simulink model "cascade_model"  (R2026a)
settings: Solver=VariableStepAuto  StopTime=75
values from neighbouring files (symbols this model uses):
  params = base    [build_params.m]    (also in determine_cost.m = build_params(struct(      'm_structure', m,      'x_thrust',; run_initial.m = rig())
undefined symbols (not defined in the file or in its folder): DiscIntNeverNeededParam
settings Model: Creator=hardik-karan  LastModifiedBy=Work

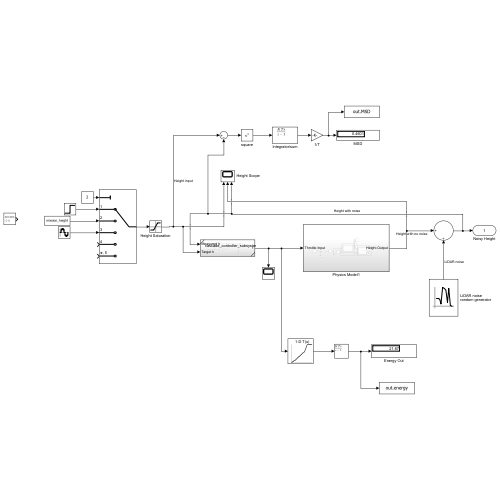
[thumbnail: Simulink's stored preview of the top-level diagram]
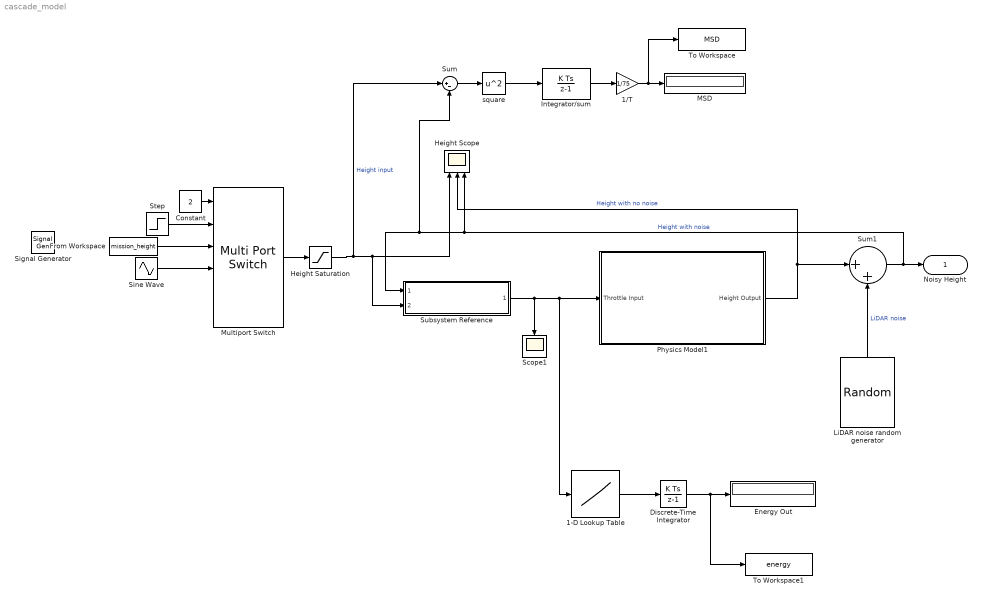
== system cascade_model ==
  1-D Lookup Table : Lookup_n-D  NumberOfTableDimensions=1  BreakpointsForDimension1=params.throttle_grid  Table=params.power_grid  InternalRulePriority=Speed  RndMeth=Simplest
  1/T : Gain  Gain=1/75
  Constant : Constant  Value=2
  Discrete-Time Integrator : DiscreteIntegrator  gainval=0.001  SampleTime=params.dt  ICPrevOutput=DiscIntNeverNeededParam  ICPrevScaledInput=DiscIntNeverNeededParam
  Energy Out : Display
      settings: Decimation=3
  From Workspace : FromWorkspace  VariableName=mission_height  SampleTime=params.dt  OutputAfterFinalValue=Holding final value
  Height Saturation : Saturate  UpperLimit=1.44  LowerLimit=0
  Height Scope : Scope  NumInputPorts=3
      settings: ActiveDisplayYMinimum=-4.73003641066337  ActiveDisplayYMaximum=6.0208709311882966  DataLoggingVariableName=ScopeData2
  Integrator/sum : DiscreteIntegrator  SampleTime=-1  ICPrevOutput=DiscIntNeverNeededParam  ICPrevScaledInput=DiscIntNeverNeededParam
  LiDAR noise random generator : RandomNumber  Variance=4.913e-05  SampleTime=params.dt
  MSD : Display
      settings: Decimation=6
  Multiport Switch : MultiPortSwitch  Inputs=5  SaturateOnIntegerOverflow=off  InputSameDT=off
  Physics Model1 : Subsystem
  Scope1 : Scope
      settings: ActiveDisplayYMinimum=-9.9999999999999982  ActiveDisplayYMaximum=90  DataLoggingVariableName=ScopeData4
  Signal Generator : SignalGenerator  Units=rad/sec
  Sine Wave : Sin  Amplitude=0.5  Bias=0.5  SampleTime=params.dt
  Step : Step  FinalValue=0.5  SampleTime=0
  Subsystem Reference : Subsystem  ReferencedSubsystem=cascade_controller_subsystem
  Sum : Sum  Inputs=|+-
  Sum1 : Sum  Inputs=|++
  To Workspace : ToWorkspace  VariableName=MSD  SaveFormat=Timeseries  SampleTime=-1
  To Workspace1 : ToWorkspace  VariableName=energy  SaveFormat=Timeseries  SampleTime=-1
  square : Math  Operator=square
  Noisy Height : Outport
  wires:
  Multiport Switch/1 -> Height Saturation/1
  Subsystem Reference/1 -> 1-D Lookup Table/1, Physics Model1/1(Throttle Input), Scope1/1
  Height Saturation/1 -> Sum/1, Subsystem Reference/2, Height Scope/1  "Height input"
  Physics Model1/1(Height Output) -> Height Scope/2, Sum1/1  "Height with no noise"
  Step/1 -> Multiport Switch/2
  Constant/1 -> Multiport Switch/1
  From Workspace/1 -> Multiport Switch/3
  Integrator/sum/1 -> 1/T/1
  1/T/1 -> To Workspace/1, MSD/1
  square/1 -> Integrator/sum/1
  Sum/1 -> square/1
  LiDAR noise random generator/1 -> Sum1/2  "LiDAR noise"
  Sum1/1 -> Subsystem Reference/1, Sum/2, Height Scope/3, Noisy Height/1  "Height with noise"
  1-D Lookup Table/1 -> Discrete-Time Integrator/1
  Discrete-Time Integrator/1 -> To Workspace1/1, Energy Out/1
  Sine Wave/1 -> Multiport Switch/4

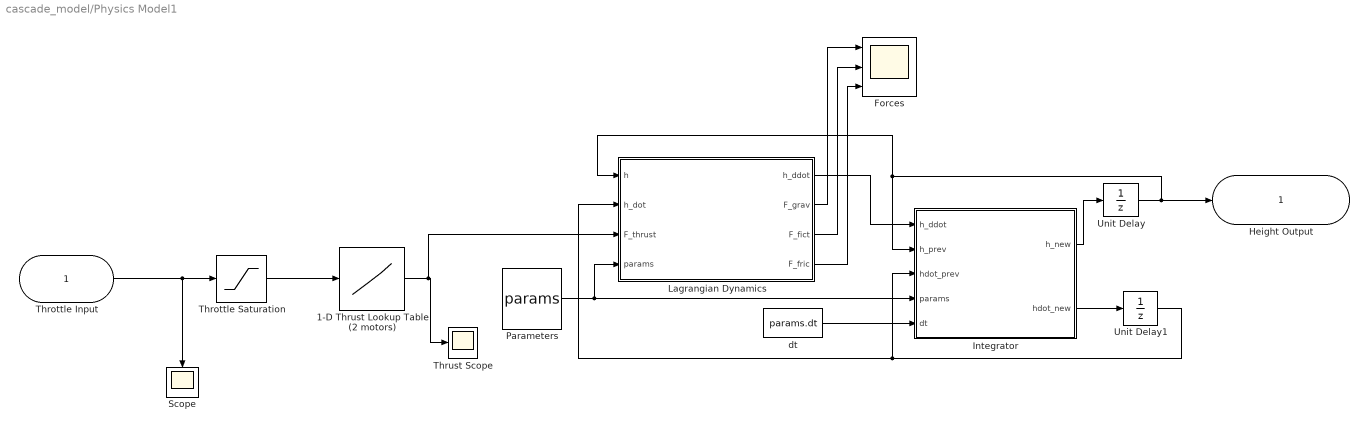
== system cascade_model/Physics Model1 ==
  Throttle Input : Inport
  " Integrator" : MATLAB Function  TreatAsAtomicUnit=on
  1-D Thrust Lookup Table (2 motors) : Lookup_n-D  NumberOfTableDimensions=1  BreakpointsForDimension1=params.throttle_grid  Table=params.thrust_grid  InternalRulePriority=Speed  RndMeth=Simplest
  Forces : Scope  NumInputPorts=3
      settings: ActiveDisplayYMinimum=-3.6083712503031267  ActiveDisplayYMaximum=10.329871439608075
  Lagrangian Dynamics : MATLAB Function  TreatAsAtomicUnit=on
  Parameters : Constant  Value=params  OutDataTypeStr=Bus: paramsBus
  Scope : Scope
      settings: ActiveDisplayYMinimum=-1.112056083934803  ActiveDisplayYMaximum=87.723110182330359  DataLoggingVariableName=ScopeData3
  Throttle Saturation : Saturate  UpperLimit=80  LowerLimit=0
  Thrust Scope : Scope
      settings: ActiveDisplayYMinimum=-6.06231372429491  ActiveDisplayYMaximum=25.225066228039402
  Unit Delay : UnitDelay  SampleTime=-1
  Unit Delay1 : UnitDelay  SampleTime=-1
  dt : Constant  Value=params.dt
  Height Output : Outport
  wires:
  Parameters/1 -> Lagrangian Dynamics/4(params), " Integrator"/4(params)
  Lagrangian Dynamics/2(F_grav) -> Forces/1
  Lagrangian Dynamics/3(F_fict) -> Forces/2
  " Integrator"/1(h_new) -> Unit Delay/1
  Throttle Saturation/1 -> 1-D Thrust Lookup Table (2 motors)/1
  1-D Thrust Lookup Table (2 motors)/1 -> Lagrangian Dynamics/3(F_thrust), Thrust Scope/1
  Unit Delay1/1 -> " Integrator"/3(hdot_prev), Lagrangian Dynamics/2(h_dot)
  Lagrangian Dynamics/1(h_ddot) -> " Integrator"/1(h_ddot)
  dt/1 -> " Integrator"/5(dt)
  Throttle Input/1 -> Scope/1, Throttle Saturation/1
  Unit Delay/1 -> Height Output/1, " Integrator"/2(h_prev), Lagrangian Dynamics/1(h)
  Lagrangian Dynamics/4(F_fric) -> Forces/3
  " Integrator"/2(hdot_new) -> Unit Delay1/1

== matlab function cascade_model/Physics Model1/ Integrator ==
  data: h_ddot input; h_new output; h_prev input; hdot_prev input; params input; dt input; hdot_new output
function [h_new, hdot_new] = integrator(h_ddot, h_prev, hdot_prev, params, dt)
    hdot_new = hdot_prev + h_ddot * dt;
    h_new = h_prev + hdot_new * dt;
    if h_new >= params.h_max && hdot_new > 0
        h_new = params.h_max; 
        hdot_new = 0;
    elseif h_new <= params.h_min && hdot_new < 0
        h_new = params.h_min; 
        hdot_new = 0;
    end
end

== matlab function cascade_model/Physics Model1/Lagrangian Dynamics ==
  data: h input; h_ddot output; h_dot input; F_thrust input; params input; F_grav output; F_fict output; F_fric output
function [h_ddot, F_grav, F_fict, F_fric] = lagrangian_dynamics(h, h_dot, F_thrust, params)
    [h_ddot, F_grav, F_fict, F_fric] = lagrangian(h, h_dot, F_thrust, params);
end
